simulink model "suspension_lqr_multibody"  (R2022b)
settings: Solver=ode15s  StartTime=0.0  StopTime=stopTime  MaxStep=0.002  RelTol=1e-8  AbsTol=1e-10
model workspace (MAT data in the model file):
  K = [0 2300000 500000000 0]
  Ki = 8000000
  Nbar = 0
  antiWindup = 0
  b1 = 350
  b2 = 15020
  k1 = 80000
  k2 = 500000
  m1 = 2500
  m2 = 320
  roadHeight = 0.1
  roadTau = 0.001
  roadTime = 0.5
  stopTime = 10
  umax = inf
undefined symbols (not defined in the file or in its folder): X, Y, Z
libraries: sm_lib x8, nesl_utility x7
settings Model: Creator=shark  LastModifiedBy=shark

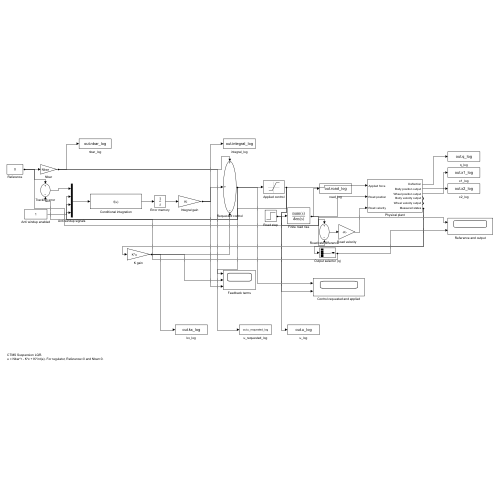
[thumbnail: Simulink's stored preview of the top-level diagram]
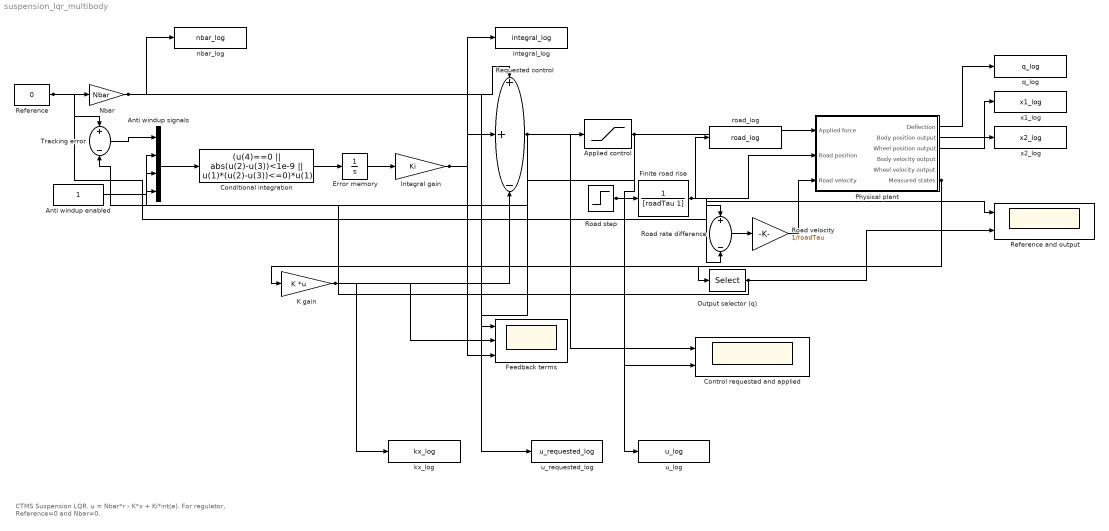
== system suspension_lqr_multibody ==
  note: CTMS Suspension LQR.
      | u = Nbar*r - K*x + Ki*int(e). For regulator, Reference=0 and Nbar=0.
  Anti windup enabled : Constant
  Anti windup signals : Mux
  Applied control : Saturate  UpperLimit=umax  LowerLimit=-umax
  Conditional integration : Fcn  Expr=(u(4)==0 || abs(u(2)-u(3))<1e-9 || u(1)*(u(2)-u(3))<=0)*u(1)
  Control requested and applied : Scope  NumInputPorts=2
  Error memory : Integrator
  Feedback terms : Scope  NumInputPorts=3
  Finite road rise : TransferFcn  Numerator=1  Denominator=[roadTau 1]
  Integral gain : Gain  Gain=Ki
  K gain : Gain  Gain=K  Multiplication=Matrix(K*u)
  Nbar : Gain  Gain=Nbar
  Output selector (q) : Selector  InputPortWidth=4  IndexOptions=Index vector (dialog)  Indices=3  OutputSizes=1
  Physical plant : Subsystem
  Reference : Constant  Value=0
  Reference and output : Scope  NumInputPorts=2
  Requested control : Sum  Inputs=++-
  Road rate difference : Sum  Inputs=+-
  Road step : Step  Time=roadTime  After=roadHeight  SampleTime=0
  Road velocity : Gain  Gain=1/roadTau
  Tracking error : Sum  Inputs=+-
  integral_log : ToWorkspace  VariableName=integral_log  SaveFormat=Timeseries  SampleTime=-1
  kx_log : ToWorkspace  VariableName=kx_log  SaveFormat=Timeseries  SampleTime=-1
  nbar_log : ToWorkspace  VariableName=nbar_log  SaveFormat=Timeseries  SampleTime=-1
  q_log : ToWorkspace  VariableName=q_log  SaveFormat=Timeseries  SampleTime=-1
  road_log : ToWorkspace  VariableName=road_log  SaveFormat=Timeseries  SampleTime=-1
  u_log : ToWorkspace  VariableName=u_log  SaveFormat=Timeseries  SampleTime=-1
  u_requested_log : ToWorkspace  VariableName=u_requested_log  SaveFormat=Timeseries  SampleTime=-1
  x1_log : ToWorkspace  VariableName=x1_log  SaveFormat=Timeseries  SampleTime=-1
  x2_log : ToWorkspace  VariableName=x2_log  SaveFormat=Timeseries  SampleTime=-1
  wires:
  Reference/1 -> Nbar/1, Tracking error/1, Reference and output/1
  Physical plant/6(Measured states) -> Output selector (q)/1, K gain/1
  Output selector (q)/1 -> Tracking error/2, Reference and output/2
  Tracking error/1 -> Anti windup signals/1
  Requested control/1 -> Anti windup signals/2, Applied control/1, Control requested and applied/1, u_requested_log/1
  Applied control/1 -> Anti windup signals/3, Physical plant/1(Applied force), Control requested and applied/2, u_log/1
  Anti windup enabled/1 -> Anti windup signals/4
  Anti windup signals/1 -> Conditional integration/1
  Conditional integration/1 -> Error memory/1
  Error memory/1 -> Integral gain/1
  Nbar/1 -> Requested control/1, Feedback terms/1, nbar_log/1
  Integral gain/1 -> Requested control/2, Feedback terms/3, integral_log/1
  K gain/1 -> Requested control/3, Feedback terms/2, kx_log/1
  Road step/1 -> Finite road rise/1, Road rate difference/1
  Finite road rise/1 -> Road rate difference/2, Physical plant/2(Road position), road_log/1
  Road rate difference/1 -> Road velocity/1
  Road velocity/1 -> Physical plant/3(Road velocity)
  Physical plant/1(Deflection) -> q_log/1
  Physical plant/2(Body position output) -> x1_log/1
  Physical plant/3(Wheel position output) -> x2_log/1

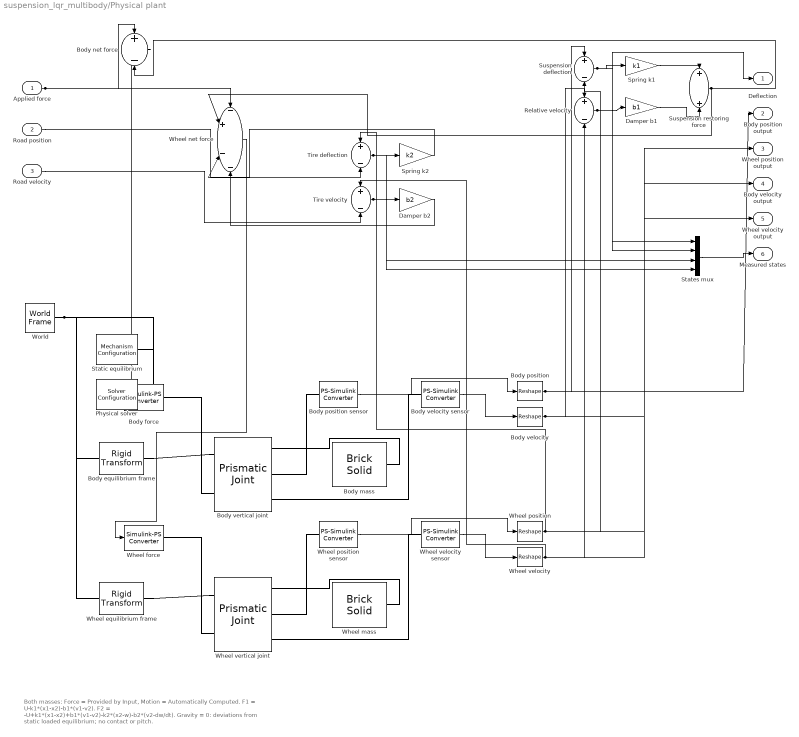
== system suspension_lqr_multibody/Physical plant ==
  note: Both masses: Force = Provided by Input, Motion = Automatically Computed.
      | F1 = U-k1*(x1-x2)-b1*(v1-v2).
      | F2 = -U+k1*(x1-x2)+b1*(v1-v2)-k2*(x2-w)-b2*(v2-dw/dt).
      | Gravity = 0: deviations from static loaded equilibrium; no contact or pitch.
  Applied force : Inport
  Road position : Inport  Port=2
  Road velocity : Inport  Port=3
  Body equilibrium frame : sm_lib/Frames and Transforms/Rigid Transform  TranslationMethod=Cartesian  TranslationStandardOffset=0  TranslationLengthUnit=m  TranslationStandardAxis=+Z  TranslationCartesianOffset=[0 0 1.4]  TranslationROffset=0  TranslationROffsetUnits=m  TranslationZOffset=0  TranslationZOffsetUnits=m  TranslationThetaOffset=0  TranslationThetaOffsetUnits=deg  RotationMethod=None  RotationAngleUnits=deg  RotationStandardAxis=+Z  RotationAngle=0.0  RotationArbitraryAxis=[0 0 1]  FollAlignAxisA=+X  BaseAlignAxisA=+Y  FollAlignAxisB=+Y  BaseAlignAxisB=+Z  RotationSequenceAxes=FollowerAxes  RotationSequence=XYX  RotationSequenceAngles=[0 0 0]  RotationSequenceAnglesUnits=deg  RotationMatrix=[1 0 0; 0 1 0; 0 0 1]  Quaternion=[1 0 0 0]
  Body force : nesl_utility/Simulink-PS Converter  PhysicalDomain=network_engine_domain  SubClassName=ps_input  LeftPortType=input  RightPortType=output  PseudoPeriodic=off  Frequencies=[]  NoiseDistribution=none  NoiseParameters=[]  Unit=N  AffineConversion=off  FilteringAndDerivatives=provide  SimscapeFilterOrder=1  InputFilterTimeConstant=0.001  UdotUserProvided=0
  Body mass : sm_lib/Body Elements/Brick Solid  GraphicAmbientColor=[0.15 0.15 0.15 1.0]  BasedOnType=Mass  BrickDimensions=[1.5 0.7 0.3]  BrickDimensionUnits=m  CenterOfMass=[0 0 0]  CenterOfMassUnits=m  GraphicDiffuseColor=[0.1 0.45 0.8]  Density=1000  DensityUnits=kg/m^3  DoExposeReferenceFrame=on  GraphicEmissiveColor=[0.0 0.0 0.0 1.0]  ExportEntireGeometry=off  SerializedFrames=<Frames/>  MarkerShape=Sphere  MarkerSize=10  GraphicType=FromGeometry  InertiaType=CalculateFromGeometry  Mass=m1  MassUnits=kg  MomentsOfInertia=[1 1 1]  MomentsOfInertiaUnits=kg*m^2  GraphicOpacity=1.0  ProductsOfInertia=[0 0 0]  ProductsOfInertiaUnits=kg*m^2  GraphicShininess=75  GraphicSpecularColor=[0.5 0.5 0.5 1.0]  GraphicVisPropType=SimpleVisualProperties
  Body net force : Sum  Inputs=+-
  Body position : Reshape
  Body position sensor : nesl_utility/PS-Simulink Converter  PhysicalDomain=network_engine_domain  SubClassName=ps_output  LeftPortType=input  RightPortType=output  PseudoPeriodic=off  Frequencies=[]  VectorFormat=inherit  Unit=m  AffineConversion=off
  Body velocity : Reshape
  Body velocity sensor : nesl_utility/PS-Simulink Converter  PhysicalDomain=network_engine_domain  SubClassName=ps_output  LeftPortType=input  RightPortType=output  PseudoPeriodic=off  Frequencies=[]  VectorFormat=inherit  Unit=m/s  AffineConversion=off
  Body vertical joint : sm_lib/Joints/Prismatic Joint  JointMode=Normal  SenseConstraintForce=off  SenseConstraintForceX=off  SenseConstraintForceY=off  SenseConstraintForceZ=off  SenseConstraintTorque=off  SenseConstraintTorqueX=off  SenseConstraintTorqueY=off  SenseConstraintTorqueZ=off  SenseTotalForce=off  SenseTotalForceX=off  SenseTotalForceY=off  SenseTotalForceZ=off  SenseTotalTorque=off  SenseTotalTorqueX=off  SenseTotalTorqueY=off  SenseTotalTorqueZ=off  CompositeWrenchDir=FollowerOnBase  CompositeWrenchFrame=BaseFrame  EquilibriumPosition=0  EquilibriumPositionUnits=m  SpringStiffness=0  SpringStiffnessUnits=N/m  DampingCoefficient=0  DampingCoefficientUnits=N/(m/s)  TorqueActuationMode=InputTorque  MotionActuationMode=ComputedMotion  SensePosition=on  SenseVelocity=on  SenseAcceleration=off  SenseTorqueForce=off  SenseLowerLimitTorqueForce=off  SenseUpperLimitTorqueForce=off  LowerLimitSpecify=off  LowerLimitBound=-1  LowerLimitBoundUnits=m  LowerLimitStiffness=1e6  LowerLimitStiffnessUnits=N/m  LowerLimitDamping=1e3  LowerLimitDampingUnits=N/(m/s)  LowerLimitTransitionRegionWidth=1e-4  LowerLimitTransitionRegionWidthUnits=m  UpperLimitSpecify=off  UpperLimitBound=1  UpperLimitBoundUnits=m  UpperLimitStiffness=1e6  UpperLimitStiffnessUnits=N/m  UpperLimitDamping=1e3  UpperLimitDampingUnits=N/(m/s)  UpperLimitTransitionRegionWidth=1e-4  UpperLimitTransitionRegionWidthUnits=m  PositionTargetSpecify=on  PositionTargetPriority=High  PositionTargetValue=0  PositionTargetValueUnits=m  VelocityTargetSpecify=on  VelocityTargetPriority=High  VelocityTargetValue=0  VelocityTargetValueUnits=m/s
  Damper b1 : Gain  Gain=b1
  Damper b2 : Gain  Gain=b2
  Physical solver : nesl_utility/Solver Configuration  PhysicalDomain=network_engine_domain  SubClassName=solver  LeftPortType=input  RightPortType=generic  Tones=[]  Harmonics=[]  SimulateNoise=off  Profile=off  UseLocalSampling=off  EnableSwitchedLinearOptims=on  FrequencyDomain=off  UseCCode=off  RelTol=0.001  AbsTol=0.001  MinStep=1e-09  ToWorkspace=off  RevertToSquareIcSolve=off  NumHomotopyIterations=100  PhasorMode=off  PhasorModeNumHarmonics=1  ConsistencySolver=NEWTON_XTOL_AFTER_FTOL  IndexReductionMethod=DerivativeReplacement  DoDC=off  ResidualTolerance=1e-09  ConsistencyTolSource=GLOBAL  ConsistencyAbsTol=0.001  ConsistencyRelTol=0.001  ConsistencyTolFactor=0.001  UseLocalSolver=off  LocalSolverChoice=NE_BACKWARD_EULER_ADVANCER  ResolveIndetEquations=on  FunctionEvalNumThread=1  LocalSolverSampleTime=0.001  DoFixedCost=off  MaxNonlinIter=3  MaxModeIter=2  ComputeImpulses=off  ImpulseIterations=2  LinearAlgebra=auto  LinearAlgebraNumThread=0  EquationFormulation=NE_TIME_EF  DelaysMemoryBudget=1024  AutomaticFiltering=on  FilteringTimeConstant=0.001  PartitionStorageMethod=AS_NEEDED  PartitionMemoryBudget=1024  PartitionMethod=ROBUST
  Relative velocity : Sum  Inputs=+-
  Spring k1 : Gain  Gain=k1
  Spring k2 : Gain  Gain=k2
  States mux : Mux
  Static equilibrium : sm_lib/Utilities/Mechanism Configuration  UniformGravity=Constant  GravityVector=[0 0 0]  GravityUnits=m/s^2  LinearizationDelta=0.001  JointModeTransitionNonlinearIterations=2
  Suspension deflection : Sum  Inputs=+-
  Suspension restoring force : Sum
  Tire deflection : Sum  Inputs=+-
  Tire velocity : Sum  Inputs=+-
  Wheel equilibrium frame : sm_lib/Frames and Transforms/Rigid Transform  TranslationMethod=Cartesian  TranslationStandardOffset=0  TranslationLengthUnit=m  TranslationStandardAxis=+Z  TranslationCartesianOffset=[0 0 0.35]  TranslationROffset=0  TranslationROffsetUnits=m  TranslationZOffset=0  TranslationZOffsetUnits=m  TranslationThetaOffset=0  TranslationThetaOffsetUnits=deg  RotationMethod=None  RotationAngleUnits=deg  RotationStandardAxis=+Z  RotationAngle=0.0  RotationArbitraryAxis=[0 0 1]  FollAlignAxisA=+X  BaseAlignAxisA=+Y  FollAlignAxisB=+Y  BaseAlignAxisB=+Z  RotationSequenceAxes=FollowerAxes  RotationSequence=XYX  RotationSequenceAngles=[0 0 0]  RotationSequenceAnglesUnits=deg  RotationMatrix=[1 0 0; 0 1 0; 0 0 1]  Quaternion=[1 0 0 0]
  Wheel force : nesl_utility/Simulink-PS Converter  PhysicalDomain=network_engine_domain  SubClassName=ps_input  LeftPortType=input  RightPortType=output  PseudoPeriodic=off  Frequencies=[]  NoiseDistribution=none  NoiseParameters=[]  Unit=N  AffineConversion=off  FilteringAndDerivatives=provide  SimscapeFilterOrder=1  InputFilterTimeConstant=0.001  UdotUserProvided=0
  Wheel mass : sm_lib/Body Elements/Brick Solid  GraphicAmbientColor=[0.15 0.15 0.15 1.0]  BasedOnType=Mass  BrickDimensions=[0.6 0.45 0.3]  BrickDimensionUnits=m  CenterOfMass=[0 0 0]  CenterOfMassUnits=m  GraphicDiffuseColor=[0.15 0.15 0.18]  Density=1000  DensityUnits=kg/m^3  DoExposeReferenceFrame=on  GraphicEmissiveColor=[0.0 0.0 0.0 1.0]  ExportEntireGeometry=off  SerializedFrames=<Frames/>  MarkerShape=Sphere  MarkerSize=10  GraphicType=FromGeometry  InertiaType=CalculateFromGeometry  Mass=m2  MassUnits=kg  MomentsOfInertia=[1 1 1]  MomentsOfInertiaUnits=kg*m^2  GraphicOpacity=1.0  ProductsOfInertia=[0 0 0]  ProductsOfInertiaUnits=kg*m^2  GraphicShininess=75  GraphicSpecularColor=[0.5 0.5 0.5 1.0]  GraphicVisPropType=SimpleVisualProperties
  Wheel net force : Sum  Inputs=-+--
  Wheel position : Reshape
  Wheel position sensor : nesl_utility/PS-Simulink Converter  PhysicalDomain=network_engine_domain  SubClassName=ps_output  LeftPortType=input  RightPortType=output  PseudoPeriodic=off  Frequencies=[]  VectorFormat=inherit  Unit=m  AffineConversion=off
  Wheel velocity : Reshape
  Wheel velocity sensor : nesl_utility/PS-Simulink Converter  PhysicalDomain=network_engine_domain  SubClassName=ps_output  LeftPortType=input  RightPortType=output  PseudoPeriodic=off  Frequencies=[]  VectorFormat=inherit  Unit=m/s  AffineConversion=off
  Wheel vertical joint : sm_lib/Joints/Prismatic Joint  JointMode=Normal  SenseConstraintForce=off  SenseConstraintForceX=off  SenseConstraintForceY=off  SenseConstraintForceZ=off  SenseConstraintTorque=off  SenseConstraintTorqueX=off  SenseConstraintTorqueY=off  SenseConstraintTorqueZ=off  SenseTotalForce=off  SenseTotalForceX=off  SenseTotalForceY=off  SenseTotalForceZ=off  SenseTotalTorque=off  SenseTotalTorqueX=off  SenseTotalTorqueY=off  SenseTotalTorqueZ=off  CompositeWrenchDir=FollowerOnBase  CompositeWrenchFrame=BaseFrame  EquilibriumPosition=0  EquilibriumPositionUnits=m  SpringStiffness=0  SpringStiffnessUnits=N/m  DampingCoefficient=0  DampingCoefficientUnits=N/(m/s)  TorqueActuationMode=InputTorque  MotionActuationMode=ComputedMotion  SensePosition=on  SenseVelocity=on  SenseAcceleration=off  SenseTorqueForce=off  SenseLowerLimitTorqueForce=off  SenseUpperLimitTorqueForce=off  LowerLimitSpecify=off  LowerLimitBound=-1  LowerLimitBoundUnits=m  LowerLimitStiffness=1e6  LowerLimitStiffnessUnits=N/m  LowerLimitDamping=1e3  LowerLimitDampingUnits=N/(m/s)  LowerLimitTransitionRegionWidth=1e-4  LowerLimitTransitionRegionWidthUnits=m  UpperLimitSpecify=off  UpperLimitBound=1  UpperLimitBoundUnits=m  UpperLimitStiffness=1e6  UpperLimitStiffnessUnits=N/m  UpperLimitDamping=1e3  UpperLimitDampingUnits=N/(m/s)  UpperLimitTransitionRegionWidth=1e-4  UpperLimitTransitionRegionWidthUnits=m  PositionTargetSpecify=on  PositionTargetPriority=High  PositionTargetValue=0  PositionTargetValueUnits=m  VelocityTargetSpecify=on  VelocityTargetPriority=High  VelocityTargetValue=0  VelocityTargetValueUnits=m/s
  World : sm_lib/Frames and Transforms/World Frame
  Deflection : Outport
  Body position output : Outport  Port=2
  Wheel position output : Outport  Port=3
  Body velocity output : Outport  Port=4
  Wheel velocity output : Outport  Port=5
  Measured states : Outport  Port=6
  wires:
  Body position sensor/1 -> Body position/1
  Body velocity sensor/1 -> Body velocity/1
  Wheel position sensor/1 -> Wheel position/1
  Wheel velocity sensor/1 -> Wheel velocity/1
  Body position/1 -> Suspension deflection/1, Body position output/1
  Wheel position/1 -> Suspension deflection/2, Wheel position output/1, Tire deflection/1
  Body velocity/1 -> Relative velocity/1, Body velocity output/1
  Wheel velocity/1 -> Relative velocity/2, Wheel velocity output/1, Tire velocity/1
  Suspension deflection/1 -> Spring k1/1, Deflection/1, States mux/1
  Relative velocity/1 -> Damper b1/1, States mux/2
  Spring k1/1 -> Suspension restoring force/1
  Damper b1/1 -> Suspension restoring force/2
  Road position/1 -> Tire deflection/2
  Road velocity/1 -> Tire velocity/2
  Tire deflection/1 -> Spring k2/1, States mux/3
  Tire velocity/1 -> Damper b2/1, States mux/4
  Applied force/1 -> Body net force/1, Wheel net force/1
  Suspension restoring force/1 -> Body net force/2, Wheel net force/2
  Spring k2/1 -> Wheel net force/3
  Damper b2/1 -> Wheel net force/4
  Body net force/1 -> Body force/1
  Wheel net force/1 -> Wheel force/1
  States mux/1 -> Measured states/1
  connections:
  Static equilibrium/RConn1 -- World/RConn1 -- Physical solver/RConn1 -- Body equilibrium frame/LConn1 -- Wheel equilibrium frame/LConn1
  Body equilibrium frame/RConn1 -- Body vertical joint/LConn1
  Body force/RConn1 -- Body vertical joint/LConn2
  Body vertical joint/RConn1 -- Body mass/RConn1
  Body vertical joint/RConn2 -- Body position sensor/LConn1
  Body vertical joint/RConn3 -- Body velocity sensor/LConn1
  Wheel equilibrium frame/RConn1 -- Wheel vertical joint/LConn1
  Wheel force/RConn1 -- Wheel vertical joint/LConn2
  Wheel vertical joint/RConn1 -- Wheel mass/RConn1
  Wheel vertical joint/RConn2 -- Wheel position sensor/LConn1
  Wheel vertical joint/RConn3 -- Wheel velocity sensor/LConn1
